simulink library "WBToolboxLibrary"  (R2014b)
settings: Solver=ode45  StartTime=0.0  StopTime=10.0  RelTol=1e-3
undefined symbols (not defined in the file): WBT_modelName, WBT_robotName, WBT_wbiFilename, WBT_wbiList
libraries: simulink x1
(part 1 of 2)
settings Model: CovSaveCumulativeToWorkspaceVar=on  Creator=jorhabib  LastModifiedBy=dferigo

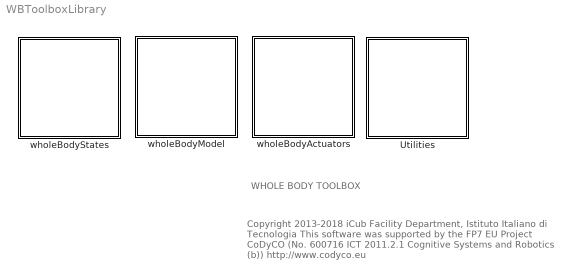
== system WBToolboxLibrary ==
  note: WHOLE BODY TOOLBOX
  note: Copyright  2013-2018 iCub Facility Department, Istituto Italiano di Tecnologia
      | This software was supported by the FP7 EU Project CoDyCO (No. 600716 ICT 2011.2.1 Cognitive Systems and Robotics (b))
      | http://www.codyco.eu
  Utilities : Subsystem
      mask Display: image(imread('utilities.png'))
  wholeBodyActuators : Subsystem
      mask Display: image(imread('wholeBodyActuators.png'),'center')
  wholeBodyModel : Subsystem
      mask Display: image(imread('wholeBodyModel.png'),'center')
  wholeBodyStates : Subsystem
      mask Display: image(imread('wholeBodyStates.png'),'center');

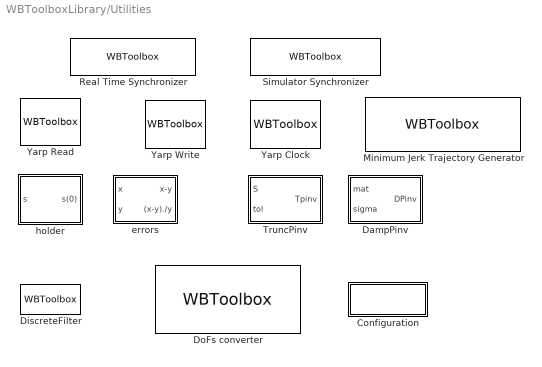
== system WBToolboxLibrary/Utilities ==
  Configuration : Subsystem  InitFcn=|  mask{ConfigSource=Mask, ConfigObject='WBTConfigRobot', RobotName='icub', UrdfFile='model.urdf', ControlledJoints={'l_elbow','l_shoulder_pitch','torso_roll'}, ControlBoardsNames={'left_arm','right_arm','torso'}, LocalName='WBT', GravityVector=[0,0,-9.81]}
      | source = get_param(gcb,'ConfigSource');
      | 
      | if strcmp(source, 'Workspace')
      |     object = get_param(gcb,'ConfigObject');
      |     WBToolbox.ConfigurationToMask(gcb, object);
      | end
      | 
      | WBToolbox.MaskToConfiguration(gcb);
      | 
      | clear object source
      mask prompts: ConfigSource "Configuration from"; ConfigObject "Name of the object"; RobotName "Robot Name"; UrdfFile "Urdf File"; ControlledJoints "Controlled Joints"; ControlBoardsNames "Control Boards Names"; LocalName "Local Name"; GravityVector "Gravity Vector"
      mask TypeOptions ConfigSource: Workspace | Mask
      mask Callback ConfigSource:
      | % Get the Workspace/Mask menu
      | h = Simulink.Mask.get(gcb);
      | currentConfigSource = get_param(gcb,'ConfigSource');
      | 
      | if strcmp(currentConfigSource,'Workspace')
      |     % Switch the visibility of the GUI elements
      |     set_param(gcb,'MaskVisibilities',{'on';'on';'on';'on';'on';'on';'on';'on';});
      |     h.Parameters(3).ReadOnly = 'on';
      |     h.Parameters(4).ReadOnly = 'on';
      |     h.Parameters(5).ReadOnly = 'on';
      |     h.Parameters(6).ReadOnly = 'on';
      |     h.Parameters(7).ReadOnly = 'on';
      |     h.Parameters(8).ReadOnly = 'on';
      | 
      |     % Parse the object inserted in the ConfigObject field
      |     currentConfigObject = get_param(gcb,'ConfigObject');
      |     WBToolbox.ConfigurationToMask(gcb,currentConfigObject);
      |     clear currentConfigObject;
      | elseif strcmp(currentConfigSource,'Mask')
      |     % Switch the visibility of the GUI elements
      |     set_param(gcb,'MaskVisibilities',{'on';'off';'on';'on';'on';'on';'on';'on';});
      |     h.Parameters(3).ReadOnly = 'off';
      |     h.Parameters(4).ReadOnly = 'off';
      |     h.Parameters(5).ReadOnly = 'off';
      |     h.Parameters(6).ReadOnly = 'off';
      |     h.Parameters(7).ReadOnly = 'off';
      |     h.Parameters(8).ReadOnly = 'off';
      |     h.Parameters(3).Enabled = 'on';
      |     h.Parameters(4).Enabled = 'on';
      |     h.Parameters(5).Enabled = 'on';
      |     h.Parameters(6).Enabled = 'on';
      |     h.Parameters(7).Enabled = 'on';
      |     h.Parameters(8).Enabled = 'on';
      | end
      | 
      | clear h currentConfigSource
      mask Callback ConfigObject:
      | % This code get called whatsoever
      | if strcmp(char(get_param(gcb,'ConfigSource')),'Mask')
      |     return
      | end
      | 
      | % Parse the object inserted in the ConfigObject field
      | currentConfigObject = get_param(gcb,'ConfigObject');
      | WBToolbox.ConfigurationToMask(gcb,currentConfigObject);
      | 
      | clear currentConfigObject;
      mask Display: disp('Config')
  DampPinv : Subsystem  mask{tol=1e-4}
      mask prompts: tol "Tolerance"
  DiscreteFilter : S-Function  FunctionName=WBToolbox  Parameters='DiscreteFilter',filterType,numCoeffs,denCoeffs,Fc,Ts,orderMedianFilter,y0,u0  SFunctionDeploymentMode=off  EnableBusSupport=off  mask(Discrete Filter){filterType=Generic, numCoeffs=[0], denCoeffs=[0], Fc=0, Ts=0, orderMedianFilter=0, initStatus=off, y0=[0], u0=[0]}
      mask prompts: filterType "Type of the filter"; numCoeffs "Numerator Coefficients*"; denCoeffs "Denominator Coefficients*"; Fc "Cut Frequency (Hz)"; Ts "Sampling time (s)"; orderMedianFilter "Order"; initStatus "Define initial conditions"; y0 "Output y0"; u0 "Input u0"
      mask help: This block wraps the Filter, FirstOrderLowPassFilter, and MedianFilter from iCub::ctrl.
      mask init:
      | filterType = get_param(gcb, 'filterType');
      | numCoeffs  = mat2str(numCoeffs);
      | denCoeffs  = mat2str(denCoeffs);
      | 
      | initStatus = get_param(gcb, 'initStatus');
      | 
      | if (strcmp(initStatus,'on'))
      |     y0 = mat2str(y0);
      |     u0 = mat2str(u0);
      | else
      |     y0 = 'none';
      |     u0 = 'none';
      | end
      | 
      | clear initStatus
      mask TypeOptions filterType: Generic | FirstOrderLowPassFilter | MedianFilter
      mask Callback filterType:
      | % From: https://it.mathworks.com/help/simulink/slref/simulink.mask-class.html
      | filterType = get_param(gcb, 'filterType');
      | initStatus = get_param(gcb, 'initStatus');
      | p = Simulink.Mask.get(gcbh);
      | howToCoeffs = p.getDialogControl('howToCoeffs');
      | 
      | %set_param(gcb, 'initStatus','off');
      | if (strcmp(initStatus,'on'))
      |     vis_init = 'on';
      | else
      |     vis_init = 'off';
      | end
      | 
      | if(strcmp(filterType, 'Generic'))
      |     set_param(gcb, 'MaskVisibilities',{'on','on','on','off','off','off','on',vis_init,vis_init});
      |     howToCoeffs.Visible = 'on';
      | elseif(strcmp(filterType, 'FirstOrderLowPassFilter'))
      |     set_param(gcb, 'MaskVisibilities',{'on','off','off','on','on','off','on',vis_init,'off'});
      |     howToCoeffs.Visible = 'off';
      | elseif(strcmp(filterType, 'MedianFilter'))
      |     set_param(gcb, 'MaskVisibilities',{'on','off','off','off','off','on','on',vis_init,'off'});
      |     howToCoeffs.Visible = 'off';
      | end
      | 
      | clear filterType initStatus p howToCoeffs vis_init;
      mask Callback initStatus:
      | initStatus   = get_param(gcb, 'initStatus');
      | visibilities = get_param(gcb, 'MaskVisibilities');
      | filterType   = get_param(gcb, 'filterType');
      | 
      | if (strcmp(initStatus,'off'))
      |     visibilities{8} = 'off';
      |     visibilities{9} = 'off';
      | elseif (strcmp(initStatus,'on'))
      |     visibilities{8} = 'on';
      |     if (strcmp(filterType,'Generic'))
      |         visibilities{9} = 'on';
      |     end
      | end
      | 
      | set_param(gcb, 'MaskVisibilities', visibilities);
      | 
      | clear initStatus visibilities filterType;
      mask DialogControl howToCoeffs Prompt: * The coefficients are ordered in increasing power of z^-1
      mask Display: disp('Filter')
  DoFs converter : S-Function  FunctionName=WBToolbox  Parameters='ModelPartitioner',WBTConfigParameters,configBlockAbsName,yarp2WBI  SFunctionDeploymentMode=off  EnableBusSupport=off  mask(DoFs converter){yarp2WBIOption=From YARP to WBI}
      mask prompts: yarp2WBIOption "Conversion Direction"
      mask help:
      | This block converts from a DoFs serialization to a YARP serialization or viceversa depending on its configuration.
      | The robot name is taken from the environment variable YARP_ROBOT_NAME.
      |
      | Parameters:
      |
      | - Conversion direction: specify if you want to convert from YARP to the current DoFs serialization or viceversa.
      mask init:
      | % WBBlock Initialization
      | % ======================
      | 
      | try
      |     [configBlockAbsName, WBTConfig] = WBToolbox.BlockInitialization(gcb, gcs);
      |     
      |     WBTConfigParameters = WBTConfig.getSimulinkParameters;
      |     clear WBTConfig;
      | catch
      | end
      | 
      | % ModelPartitioner Initialization
      | % ===============================
      | 
      | switch get_param(gcb, 'yarp2WBIOption')
      |     case 'From YARP to WBI'
      |         yarp2WBI = true;
      |     case 'From WBI to YARP'
      |         yarp2WBI = false;
      |     otherwise
      | end
      mask TypeOptions yarp2WBIOption: From YARP to WBI | From WBI to YARP
      mask DialogControl toggleHighlighting Prompt: Toggle Config Block Highlighting
      mask DialogControl toggleHighlighting Callback:
      | [configBlock, ~] = WBToolbox.BlockInitialization(gcb, gcs);
      | 
      | try
      |     if (strcmp(get_param(configBlock,'HiliteAncestors'),'none'))
      |         hilite_system(configBlock,'find');
      |     else
      |         hilite_system(configBlock,'none');
      |     end
      | catch
      |     error('[%s:ShowConfigBlock:Callback] Failed to process config block name: %s',gcb,configBlock);
      | end
      | 
      | clear configBlock
      mask Display:
      | robotName = getenv('YARP_ROBOT_NAME');
      | 
      | currentSelection = get_param(gcb,'yarp2WBIoption');
      | 
      | if strcmp(currentSelection,'From YARP to WBI')
      |     direction = 'YARP -> DoFs';
      | else
      |     direction = 'DoFs -> YARP';
      | end
      | 
      | fprintf('%s\n\n%s', robotName, direction);
  Minimum Jerk Trajectory Generator : S-Function  FunctionName=WBToolbox  Parameters='MinimumJerkTrajectoryGenerator',sampleTime, settlingTime, firstDerivatives, secondDerivatives, explicitInitialValue, externalSettlingTime,resetOnSettlingTime  SFunctionDeploymentMode=off  EnableBusSupport=off  mask(Minimum Jerk Trajectory Generator){externalSettlingTime=off, settlingTime=3, sampleTime=0.01, resetOnSettlingTime=off, firstDerivatives=on, secondDerivatives=on, explicitInitialValue=off}
      mask prompts: externalSettlingTime "External Settling Time"; settlingTime "Settling Time"; sampleTime "Sample Time"; resetOnSettlingTime "Reset on Settling Time Changes"; firstDerivatives "Output First Derivative"; secondDerivatives "Output Second Derivative"; explicitInitialValue "Explicit Initial Value"
      mask help:
      | This block wraps the minJerkTrajGen class from iCub::ctrl::minJerkTrajGen.
      |
      | The Minimum Jerk Trajectory Generator is approximated using a
      | 3rd order LTI dynamical system
      | (for more details see [1]).
      | Position, velocity and acceleration trajectories are computed.
      |  The main advantage with respect to the standard polynomial
      | form is that if the reference value yd changes
      | there is no need to recompute the filter coefficients.
      |
      | [1] Pattacini, U.; Nori, F.; Natale, L.; Metta, G.; Sandini, G., "An experimental evaluation of a novel minimum-jerk cartesian controller for humanoid robots," in Intelligent Robots and Systems (IROS), 2010 IEEE/RSJ International Conference on , vol., no., pp.1668-1674, 18-22 Oct. 2010
      | doi: 10.1109/IROS.2010.5650851
      | URL: http://ieeexplore.ieee.org/stamp/stamp.jsp?tp=&arnumber=5650851&isnumber=5648787
      mask Callback externalSettlingTime:
      | externalSettlingTime = get_param(gcb, 'externalSettlingTime');
      | visibility = get_param(gcb, 'MaskVisibilities');
      | if(strcmp(externalSettlingTime, 'on'))
      |     visibility{2} = 'off';
      |     visibility{4} = 'on';
      | else
      |     visibility{2} = 'on';
      |     visibility{4} = 'off';
      | end
      | set_param(gcb, 'MaskVisibilities',visibility);
      | clear externalSettlingTime
      mask Display:
      | firstDer = get_param(gcb, 'firstDerivatives');
      | secondDer = get_param(gcb, 'secondDerivatives');
      | initialValues = get_param(gcb, 'explicitInitialValue');
      | externalSettlingTimeParam = get_param(gcb, 'externalSettlingTime');
      | 
      | %Inputs
      | portIndex = 2;
      | port_label('input', 1, 'Reference')
      | if(strcmp(initialValues, 'on'))
      |     port_label('input', portIndex, 'Initial Value')
      |     portIndex = portIndex + 1;
      | end
      | 
      | if(strcmp(externalSettlingTimeParam, 'on'))
      |     port_label('input', portIndex, 'Settling Time')
      |     portIndex = portIndex + 1;
      | end
      | 
      | %Outputs
      | port_label('output', 1, 'Signal')
      | secondDerPortIndex = 2;
      | if(strcmp(firstDer, 'on'))
      |     port_label('output', 2, 'First Derivative')
      |     secondDerPortIndex = secondDerPortIndex + 1;
      | end
      | if(strcmp(secondDer, 'on'))
      |     port_label('output', secondDerPortIndex, 'Second Derivative')
      | end
  Real Time Synchronizer : S-Function  FunctionName=WBToolbox  Parameters='RealTimeSynchronizer',period  SFunctionDeploymentMode=off  EnableBusSupport=off  mask(Real Time Synchronizer){period=0.01}
      mask prompts: period "Controller Period (in seconds)"
      mask help:
      | This block slows down the simulation trying to match the period specified
      | as parameter (in seconds).
      | The bigger the period the more probable
      | is that Simulink can remain synched with it.
      mask Display: disp('Real Time Synchronizer')
  Simulator Synchronizer : S-Function  FunctionName=WBToolbox  Parameters='SimulatorSynchronizer',period, serverPortName, clientPortName  SFunctionDeploymentMode=off  EnableBusSupport=off  mask(Simulator Synchronizer){period=0.01, serverPortName='/clock/rpc', clientPortName='/WBT_synchronizer/rpc:o'}
      mask prompts: period "Controller Period (in seconds)"; serverPortName "Server Port Name"; clientPortName "Client Port Name"
      mask help:
      | This block synchronizes with the external simulation on a simulator
      | (only Gazebo is supported at the moment).
      mask Display: disp('Simulator Synchronizer')
  TruncPinv : Subsystem  mask{tol=1e-4}
      mask prompts: tol "Tolerance"
  Yarp Clock : S-Function  FunctionName=WBToolbox  Parameters='YarpClock'  SFunctionDeploymentMode=off  EnableBusSupport=off  mask(YARP Clock){}
      mask help:
      | This block outputs the current YARP Time.
      | In a nutshell, this block outputs the equivalent of the C++ function call yarp::os::Time::now()
      mask Display: disp('YARP Time')
  Yarp Read : S-Function  FunctionName=WBToolbox  Parameters='YarpRead',portName,signalSize,blocking,timestamp,autoconnect,errorOnConnection,timeout  SFunctionDeploymentMode=off  EnableBusSupport=off  mask(YARP Read){portName='/portname', signalSize=1, timeout=0.5, blocking=off, timestamp=on, autoconnect=on, errorOnConnection=on}
      mask prompts: portName "Source Port Name"; signalSize "Port Size"; blocking "Blocking Read"; timestamp "Read Timestamp"; errorOnConnection "Error on missing connection"
      mask help:
      | This block behaves as the command 'yarp read'.
      |
      | By default it has the option 'Autoconnect' active, which means that the user can only specify the name of the port ('Source Port Name') from which readings are desired, along with the size of the expected data (e.g. 3 when reading the torso state).
      |
      | When the user unchecks 'Autoconnect', 'Opened Port Name' field shows up and it corresponds to the name of the port the block will create. No autoconnection is performed, and the output will be always zero until the user connects it to some other port from command line using 'yarp connect [from] [dest]'.
      |
      | When 'Autoconnect' is off, an additional output called 'signal' is added to the block. It outputs 1 if the port has received at least one sample, or 0 otherwise.
      mask Callback blocking:
      | blocking_val = get_param(gcb, 'blocking');
      | mask_visibility = get_param(gcb, 'MaskVisibilities');
      | 
      | if(strcmp(blocking_val, 'on'))
      |     mask_visibility{3} = 'on';
      |     set_param(gcb, 'MaskVisibilities', mask_visibility);
      | else
      |     mask_visibility{3} = 'off';
      |     set_param(gcb, 'MaskVisibilities', mask_visibility);
      | end
      | 
      | clear blocking_val mask_visibility
      mask Callback autoconnect:
      | autoconnect_val = get_param(gcb, 'Autoconnect');
      | prompt_string = get_param(gcb, 'MaskPrompts');
      | mask_visibilities = get_param(gcb, 'MaskVisibilities');
      | 
      | if(strcmp(autoconnect_val, 'on'))
      |     prompt_string{1} = 'Source Port Name';
      |     mask_visibilities{7} = 'on';
      |     set_param(gcb, 'MaskVisibilities',mask_visibilities);
      | else
      |     prompt_string{1} = 'Opened Port Name';
      |     mask_visibilities{7} = 'off';
      |     set_param(gcb, 'MaskVisibilities',mask_visibilities);
      | end
      | set_param(gcb, 'MaskPrompts', prompt_string);
      | clear autoconnect_val prompt_string mask_visibilities
      mask Display:
      | port_label('output', 1, 'signal');
      | portNumber = 1;
      | if (timestamp)
      |     portNumber = portNumber + 1;
      |     port_label('output', portNumber, 'timestamp');
      | end
      | 
      | if (~autoconnect)
      |     portNumber = portNumber + 1;
      |     port_label('output', portNumber, 'status');
      | end
  Yarp Write : S-Function  FunctionName=WBToolbox  Parameters='YarpWrite',portName,autoconnect,errorOnConnection  SFunctionDeploymentMode=off  EnableBusSupport=off  mask(YARP Write){portName='/portname', autoconnect=off, errorOnConnection=on}
      mask prompts: portName "Opened Port Name"; errorOnConnection "Error on missing connection"
      mask help:
      | This block behaves as the command 'yarp write'.
      |
      | By default this block opens a port names as the "Opened Port Name" parameter
      | and stream the input signal to that port.
      | If the option "Autoconnect" is specified, the first parameter become the
      | name of the target port to which the data will be stramed,
      | e.g. like "yarp write ... /destinationPort"
      mask Callback autoconnect:
      | autoconnect_val = get_param(gcb, 'Autoconnect');
      | prompt_string = get_param(gcb, 'MaskPrompts');
      | if(strcmp(autoconnect_val, 'on'))
      |     prompt_string{1} = 'Destination Port Name';
      |     set_param(gcb, 'MaskVisibilities',{'on';'on';'on'});
      | else
      |     prompt_string{1} = 'Opened Port Name';
      |     set_param(gcb, 'MaskVisibilities',{'on';'on';'off'});
      | end
      | set_param(gcb, 'MaskPrompts', prompt_string);
      | clear autoconnect_val prompt_string
      mask Display: disp('Yarp Write')
  errors : Subsystem  mask(Errors){}
      mask help:
      | Computes two kinds of errors. The first is just the difference between x
      | and y while the second is the ratio (x-y)/y.
  "holder " : Subsystem  mask(Holder){}
      mask help: This block holds the first input value during the simulation.

== system WBToolboxLibrary/wholeBodyActuators ==
  Set LowLevel PIDs : Subsystem  mask(Set Low Level PIDs){WBTPIDConfigObjectName='', pidType=Position}
      mask prompts: WBTPIDConfigObjectName "WBTPIDConfig Object Name"; pidType "PID Type"
      mask help:
      | This block sets the low level PID values of the controlled joints.
      |
      | The PIDs can be stored in a WBToolbox.PIDConfiguration object, each of them constructed from the WBToolbox.PID class.
      | If the number of PIDs does not match the DoFs of the Configuration block pointed by this SetLowLevelPID block, the default values are used.
      |
      | Parameters:
      | - WBToolbox.PIDConfiguration Object Name: The name of the object which store the PIDs. It must be loaded in the workspace before the simulation runs
      | - PID Type: the type of the target PIDs to set
      mask init:
      | % WBBlock Initialization
      | % ======================
      | 
      | try
      |     [configBlockAbsName, WBTConfig] = WBToolbox.BlockInitialization(gcb, gcs);
      |     
      |     WBTConfigParameters = WBTConfig.getSimulinkParameters;
      |     clear WBTConfig;
      | catch
      | end
      | 
      | % SetLowLevelPIDs Initialization
      | % ==============================
      | 
      | try
      |     PIDObjectName = WBTPIDConfigObjectName;
      |    
      |     % Remove the apices if present
      |     if (PIDObjectName(1) == "'" && ...
      |         PIDObjectName(end) == "'")
      |         PIDObjectName = PIDObjectName(2:end-1);
      |     end
      | 
      |     % Get the struct from the class
      |     PIDs = evalin('base', PIDObjectName);
      |     if (isa(PIDs,'WBToolbox.PIDConfiguration'))
      |         WBTPIDConfigStruct = PIDs.getSimulinkParameters;
      |     end
      | end
      mask TypeOptions pidType: Position | Torque
      mask Callback pidType:
      | % Get the mask parameter values. This is a cell
      | %   array of strings.
      | maskStr = get_param(gcb,'pidType');
      | 
      | switch maskStr
      |     case 'Position'
      |         set_param(gcb,'BackgroundColor', '[0.5137, 0.8510, 0.6706, 1.0]');
      |     case 'Position Direct'
      |         set_param(gcb,'BackgroundColor', '[0.3922, 0.7882, 0.3451, 1.0]');
      |     case 'Velocity'
      |         set_param(gcb,'BackgroundColor', '[0.5137, 0.6745, 1.0000, 1.0]');
      |     case 'Torque'
      |         set_param(gcb,'BackgroundColor', '[0.8275, 0.5765, 0.6039, 1.0]');
      |     otherwise
      |         error('PID Type not recognized');
      | end
      | 
      | clear  maskStr
      mask DialogControl toggleHighlighting Prompt: Toggle Config Block Highlighting
      mask DialogControl toggleHighlighting Callback:
      | [configBlock, ~] = WBToolbox.BlockInitialization(gcb, gcs);
      | 
      | try
      |     if (strcmp(get_param(configBlock,'HiliteAncestors'),'none'))
      |         hilite_system(configBlock,'find');
      |     else
      |         hilite_system(configBlock,'none');
      |     end
      | catch
      |     error('[%s:ShowConfigBlock:Callback] Failed to process config block name: %s',gcb,configBlock);
      | end
      | 
      | clear configBlock
      mask Display:
      | pidType = get_param(gcb,'pidType');
      | description = sprintf('Set Low Level\n%s PIDs', pidType);
      | disp(description);
  Set References : Subsystem  mask(Set References){controlType=Position, refSpeed=50}
      mask prompts: controlType "Control Mode"; refSpeed "Reference Speed"
      mask help:
      | This block sets the references for the robot actuators.
      | The type of control mode is specified as a parameter in the block.
      |
      | Assuming DoFs is the number of degrees of freedom configured in the Config block associated:
      |
      | Input:
      | - References: Vector of size DoFs, representing the references to be sent to the robot controlled joints.
      | - Reference Speed (Position): Set the reference speed used by the trajectory generator of the IPositionControl interface
      |
      | Parameters:
      | - Control Mode: The control mode. Choose one of the supplied mode.
      mask init:
      | % WBBlock Initialization
      | % ======================
      | 
      | try
      |     [configBlockAbsName, WBTConfig] = WBToolbox.BlockInitialization(gcb, gcs);
      |     
      |     WBTConfigParameters = WBTConfig.getSimulinkParameters;
      |     clear WBTConfig;
      | catch
      | end
      mask TypeOptions controlType: Position | Position Direct | Velocity | Torque | Open Loop | PWM | Current
      mask Callback controlType:
      | % Get the mask parameter values. This is a cell
      | %   array of strings.
      | 
      | maskStr = get_param(gcb,'controlType');
      | 
      | switch maskStr
      |     case 'Position'
      |         set_param(gcb,'BackgroundColor', '[0.5137, 0.8510, 0.6706, 1.0]');
      |         set_param(gcb,'MaskVisibilities', {'on';'on'});
      |     case 'Position Direct'
      |         set_param(gcb,'BackgroundColor', '[0.3922, 0.7882, 0.3451, 1.0]');
      |         set_param(gcb,'MaskVisibilities', {'on';'off'});
      |     case 'Velocity'
      |         set_param(gcb,'BackgroundColor', '[0.5137, 0.6745, 1.0000, 1.0]');
      |         set_param(gcb,'MaskVisibilities', {'on';'off'});
      |     case 'Torque'
      |         set_param(gcb,'BackgroundColor', '[0.8275, 0.5765, 0.6039, 1.0]');
      |         set_param(gcb,'MaskVisibilities', {'on';'off'});
      |     case 'Open Loop'
      |         set_param(gcb,'BackgroundColor', '[0.98, 0.98, 0.98, 1.0]');
      |         set_param(gcb,'MaskVisibilities', {'on';'off'});
      |     case 'PWM'
      |         set_param(gcb,'BackgroundColor', '[1, 1, 1, 1.0]');
      |         set_param(gcb,'MaskVisibilities', {'on';'off'});
      |     case 'Current'
      |         set_param(gcb,'BackgroundColor', '[0.96, 0.77, 0.46, 1.0]');
      |         set_param(gcb,'MaskVisibilities', {'on';'off'});
      |     otherwise
      |         error('Control Type not recognized.')
      | end
      | 
      | clear  maskStr
      mask DialogControl toggleHighlighting Prompt: Toggle Config Block Highlighting
      mask DialogControl toggleHighlighting Callback:
      | [configBlock, ~] = WBToolbox.BlockInitialization(gcb, gcs);
      | 
      | try
      |     if (strcmp(get_param(configBlock,'HiliteAncestors'),'none'))
      |         hilite_system(configBlock,'find');
      |     else
      |         hilite_system(configBlock,'none');
      |     end
      | catch
      |     error('[%s:ShowConfigBlock:Callback] Failed to process config block name: %s',gcb,configBlock);
      | end
      | 
      | clear configBlock
      mask Display:
      | disp(get_param(gcb,'controlType'))
      | %port_label('input',1,'References')

== system WBToolboxLibrary/wholeBodyModel ==
  Dynamics : Subsystem
      mask Display: image(imread('Dynamics.png'))
  Jacobians : Subsystem
      mask Display: image(imread('jacobian.png'))
  Kinematics : Subsystem
      mask Display: image(imread('forwardKinematics.png'))

== system WBToolboxLibrary/wholeBodyStates ==
  Get Limits : Subsystem  mask(Get Limits){limitsSource=ControlBoard, limitsType=Position}
      mask prompts: limitsSource "Limits Source"; limitsType "Limits Type"
      mask help:
      | This block provides the joint limits gathering data from either the Robot's Control Board or URDF model.
      |
      | Output:
      |
      | * Max: 1xDoFs vector containing the maximum limit
      | * Min:  1xDoFs vector containing the maximum limit
      |
      | Measures are in radians.
      mask init:
      | % WBBlock Initialization
      | % ======================
      | 
      | try
      |     [configBlockAbsName, WBTConfig] = WBToolbox.BlockInitialization(gcb, gcs);
      |     
      |     WBTConfigParameters = WBTConfig.getSimulinkParameters;
      |     clear WBTConfig;
      | catch
      | end
      | 
      | % GetLimits Initialization
      | % =========================
      | 
      | sourceLimit = get_param(gcb,'limitsSource');
      | typeLimit = get_param(gcb,'limitsType');
      | notifyError = false;
      | 
      | switch sourceLimit
      |     case 'ControlBoard'
      |         switch typeLimit
      |             case 'Position'
      |                 limitsType = 'ControlBoardPosition';
      |             case 'Velocity'
      |                 limitsType = 'ControlBoardVelocity';
      |             otherwise
      |                 notifyError = true;
      |         end
      |     case 'URDF'
      |         switch typeLimit
      |             case 'Position'
      |                 limitsType = 'ModelPosition';
      |             otherwise
      |                 notifyError = true;
      |         end
      | end
      | 
      | if notifyError
      |     error('Limit Type not recognized');
      | end
      | 
      | clear sourceLimit typeLimit notifyError
      mask TypeOptions limitsSource: ControlBoard | URDF
      mask Callback limitsSource:
      | sourceLimit = get_param(gcb,'limitsSource');
      | blockParameters = Simulink.Mask.get(gcb).Parameters;
      | limitsTypeBlockParam = blockParameters(2);
      | 
      | switch sourceLimit
      |     case 'ControlBoard'
      |         limitsTypeBlockParam.TypeOptions = {'Position','Velocity'};
      |         %limitsTypeBlockParam.Value = limitsTypeBlockParam.TypeOptions{1};
      |     case 'URDF'
      |         limitsTypeBlockParam.TypeOptions = {'Position'};
      |         %limitsTypeBlockParam.Value = limitsTypeBlockParam.TypeOptions{1};
      |     otherwise
      |         error('Limit Source not recognized');
      | end
      | 
      | clear sourceLimit blockParameters limitsTypeBlockParam
      mask TypeOptions limitsType: Position | Velocity
      mask Callback limitsType:
      | % Get the mask parameter values. This is a cell array of strings.
      | %
      | maskStr = get_param(gcb,'limitsType');
      | if strcmp(maskStr, 'Position')
      |     set_param(gcb,'BackgroundColor', '[0.5137, 0.8510, 0.6706, 1.0]');
      | elseif strcmp(maskStr, 'Velocity')
      |     set_param(gcb,'BackgroundColor', '[0.5137, 0.6745, 1.0000, 1.0]');
      | elseif strcmp(maskStr, 'Acceleration')
      |     set_param(gcb,'BackgroundColor', '[0.9255, 0.8706, 0.1333, 1.0]');
      | elseif strcmp(maskStr, 'Torque')
      |     set_param(gcb,'BackgroundColor', '[0.8275, 0.5765, 0.6039, 1.0]');
      | end
      | clear  maskStr
      mask DialogControl toggleHighlighting Prompt: Toggle Config Block Highlighting
      mask DialogControl toggleHighlighting Callback:
      | [configBlock, ~] = WBToolbox.BlockInitialization(gcb, gcs);
      | 
      | try
      |     if (strcmp(get_param(configBlock,'HiliteAncestors'),'none'))
      |         hilite_system(configBlock,'find');
      |     else
      |         hilite_system(configBlock,'none');
      |     end
      | catch
      |     error('[%s:ShowConfigBlock:Callback] Failed to process config block name: %s',gcb,configBlock);
      | end
      | 
      | clear configBlock
      mask Display:
      | fprintf('%s\n(%s)',get_param(gcb,'limitsType'),get_param(gcb,'limitsSource'))
      | 
      | port_label('output',1,'Min')
      | port_label('output',2,'Max')
  Get Measurement : Subsystem  mask(Get Measurement){measuredType=Joints Position}
      mask prompts: measuredType "Estimate Type"
      mask help:
      | This block gathers the measurement of the specified type.
      |
      | Assuming DoFs is the number of degrees of freedom of the robot,
      |
      | Output:
      | * References: Vector of size DoFs, representing the requested measurement.
      |
      | Parameters:
      | * Control Mode: The control mode. Choose one of the supplied mode.
      mask init: same as WBToolboxLibrary/wholeBodyActuators/Set References
      mask TypeOptions measuredType: Joints Position | Joints Velocity | Joints Acceleration | Joints Torque
      mask Callback measuredType:
      | % Get the mask parameter values. This is a cell
      | %   array of strings.
      | 
      | maskStr = get_param(gcb,'measuredType');
      | if strcmp(maskStr, 'Joints Position')
      |     set_param(gcb,'BackgroundColor', '[0.5137, 0.8510, 0.6706, 1.0]');
      | elseif strcmp(maskStr, 'Joints Velocity')
      |     set_param(gcb,'BackgroundColor', '[0.5137, 0.6745, 1.0000, 1.0]');
      | elseif strcmp(maskStr, 'Joints Acceleration')
      |     set_param(gcb,'BackgroundColor', '[0.9255, 0.8706, 0.1333, 1.0]');
      | elseif strcmp(maskStr, 'Joints Torque')
      |     set_param(gcb,'BackgroundColor', '[0.8275, 0.5765, 0.6039, 1.0]');
      | end
      | clear  maskStr
      mask DialogControl toggleHighlighting Prompt: Toggle Config Block Highlighting
      mask DialogControl toggleHighlighting Callback:
      | [configBlock, ~] = WBToolbox.BlockInitialization(gcb, gcs);
      | 
      | try
      |     if (strcmp(get_param(configBlock,'HiliteAncestors'),'none'))
      |         hilite_system(configBlock,'find');
      |     else
      |         hilite_system(configBlock,'none');
      |     end
      | catch
      |     error('[%s:ShowConfigBlock:Callback] Failed to process config block name: %s',gcb,configBlock);
      | end
      | 
      | clear configBlock
      mask Display: port_label('output', 1, get_param(gcb,'measuredType'))

== system WBToolboxLibrary/Utilities/Configuration ==
  ImConfig : Constant  Value=0
  Terminator : Terminator
  wires:
  ImConfig/1 -> Terminator/1

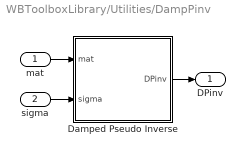
== system WBToolboxLibrary/Utilities/DampPinv ==
  mat : Inport
  sigma : Inport  Port=2
  Damped Pseudo Inverse : MATLAB Function  TreatAsAtomicUnit=on
      settings: PermitHierarchicalResolution=ParametersOnly
  DPinv : Outport
  wires:
  sigma/1 -> Damped Pseudo Inverse/2(sigma)
  Damped Pseudo Inverse/1(DPinv) -> DPinv/1
  mat/1 -> Damped Pseudo Inverse/1(mat)

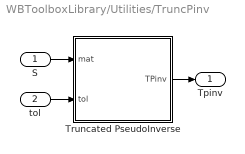
== system WBToolboxLibrary/Utilities/TruncPinv ==
  S : Inport
  tol : Inport  Port=2
  Truncated PseudoInverse : MATLAB Function  TreatAsAtomicUnit=on
      settings: PermitHierarchicalResolution=ParametersOnly
  Tpinv : Outport
  wires:
  S/1 -> Truncated PseudoInverse/1(mat)
  Truncated PseudoInverse/1(TPinv) -> Tpinv/1
  tol/1 -> Truncated PseudoInverse/2(tol)

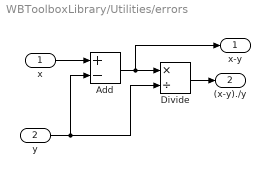
== system WBToolboxLibrary/Utilities/errors ==
  x : Inport
  y : Inport  Port=2
  Add : Sum  Inputs=+-
  Divide : Product  Inputs=*/
  x-y : Outport
  (x-y)./y : Outport  Port=2
  wires:
  Add/1 -> Divide/1, x-y/1
  x/1 -> Add/1
  y/1 -> Add/2, Divide/2
  Divide/1 -> (x-y)./y/1

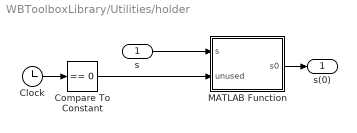
== system WBToolboxLibrary/Utilities/holder  ==
  s : Inport
  Clock : Clock
  Compare To Constant : simulink/Logic and Bit Operations/Compare To Constant  relop===  const=0  OutDataTypeStr=boolean
  MATLAB Function : MATLAB Function  TreatAsAtomicUnit=on
      settings: PermitHierarchicalResolution=ParametersOnly
  s(0) : Outport
  wires:
  Clock/1 -> Compare To Constant/1
  MATLAB Function/1(s0) -> s(0)/1
  s/1 -> MATLAB Function/1(s)
  Compare To Constant/1 -> MATLAB Function/2(unused)

== system WBToolboxLibrary/wholeBodyActuators/Set LowLevel PIDs ==
  S-Function : S-Function  FunctionName=WBToolbox  Parameters='SetLowLevelPID',WBTConfigParameters,configBlockAbsName,WBTPIDConfigStruct,pidType  SFunctionDeploymentMode=off  EnableBusSupport=off

== system WBToolboxLibrary/wholeBodyActuators/Set References ==
  References : Inport
  S-Function : S-Function  FunctionName=WBToolbox  Parameters='SetReferences',WBTConfigParameters,configBlockAbsName,controlType,refSpeed  SFunctionDeploymentMode=off  EnableBusSupport=off
  wires:
  References/1 -> S-Function/1

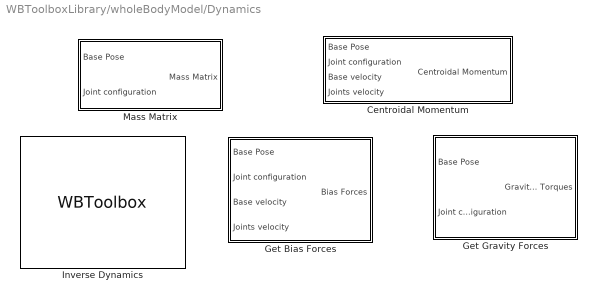
== system WBToolboxLibrary/wholeBodyModel/Dynamics ==
  Centroidal Momentum : Subsystem  mask(Centroidal Momentum){}
      mask help:
      | This block computed the 6 element centroidal momentum, as defined in:
      | "Centroidal dynamics of a humanoid robot" - DE Orin, A Goswami, SH Lee -
      | Autonomous Robots 35 (2-3), 161-176
      |
      | Assuming DoFs is the number of degrees of freedom of the robot:
      |
      | Input:
      | - Base pose: 4x4 matrix representing the homogenous transformation between the base frame and the world frame.
      | - Joint configuration: Vector of size DoFs, representing the configuration of the joints.
      | - Base velocity: Vector of size 6 representing the linear and angular velocity of the base frame.
      | - Joints velocity: Vector of size DoFs, representing the velocity of the joints.
      |
      | Output:
      | - Centroidal Momentum: 6-element vector containg the centroidal momentum (3 value for linear momentum and 3 for angular momentum)
      mask init: same as WBToolboxLibrary/wholeBodyActuators/Set References
      mask DialogControl toggleHighlighting Prompt: Toggle Config Block Highlighting
      mask DialogControl toggleHighlighting Callback:
      | [configBlock, ~] = WBToolbox.BlockInitialization(gcb, gcs);
      | 
      | try
      |     if (strcmp(get_param(configBlock,'HiliteAncestors'),'none'))
      |         hilite_system(configBlock,'find');
      |     else
      |         hilite_system(configBlock,'none');
      |     end
      | catch
      |     error('[%s:ShowConfigBlock:Callback] Failed to process config block name: %s',gcb,configBlock);
      | end
      | 
      | clear configBlock
  Get Bias Forces : Subsystem  mask(Get Generalized Bias Forces){}
      mask help:
      | This block retrieves the generalied bias forces of the robot.
      |
      | Assuming DoFs is the number of degrees of freedom of the robot:
      |
      | Input:
      | - Base pose: 4x4 matrix representing the homogenous transformation between the base frame and the world frame.
      | - Joint configuration: Vector of size DoFs, representing the configuration of the joints.
      | - Base velocity: Vector of size 6 representing the linear and angular velocity of the base frame.
      | - Joints velocity: Vector of size DoFs, representing the velocity of the joints.
      |
      | Output:
      | - Bias Forces: a Dofs + 6 vector representing the generalized bias forces of the robot.
      mask init: same as WBToolboxLibrary/wholeBodyActuators/Set References
      mask DialogControl toggleHighlighting Prompt: Toggle Config Block Highlighting
      mask DialogControl toggleHighlighting Callback:
      | [configBlock, ~] = WBToolbox.BlockInitialization(gcb, gcs);
      | 
      | try
      |     if (strcmp(get_param(configBlock,'HiliteAncestors'),'none'))
      |         hilite_system(configBlock,'find');
      |     else
      |         hilite_system(configBlock,'none');
      |     end
      | catch
      |     error('[%s:ShowConfigBlock:Callback] Failed to process config block name: %s',gcb,configBlock);
      | end
      | 
      | clear configBlock
  Get Gravity Forces : Subsystem  mask(Gravity bias){}
      mask help:
      | This block compute the generalized bias forces due to the gravity
      |
      | Assuming DoFs is the number of degrees of freedom of the robot:
      |
      | Input:
      | - Base pose: 4x4 matrix representing the homogenous transformation between the base frame and the world frame.
      | - Joint configuration: Vector of size DoFs, representing the configuration of the joints.
      |
      | Output:
      | - Gravity: a Dofs + 6 vector representing the torques due to the gravity.
      mask init: same as WBToolboxLibrary/wholeBodyActuators/Set References
      mask DialogControl toggleHighlighting Prompt: Toggle Config Block Highlighting
      mask DialogControl toggleHighlighting Callback:
      | [configBlock, ~] = WBToolbox.BlockInitialization(gcb, gcs);
      | 
      | try
      |     if (strcmp(get_param(configBlock,'HiliteAncestors'),'none'))
      |         hilite_system(configBlock,'find');
      |     else
      |         hilite_system(configBlock,'none');
      |     end
      | catch
      |     error('[%s:ShowConfigBlock:Callback] Failed to process config block name: %s',gcb,configBlock);
      | end
      | 
      | clear configBlock
  Inverse Dynamics : S-Function  FunctionName=WBToolbox  Parameters='InverseDynamics',WBTConfigParameters,configBlockAbsName  SFunctionDeploymentMode=off  EnableBusSupport=off  mask(Inverse Dynamics){}
      mask help:
      | This block compute the inverse dynamics of the robot.
      |
      | Assuming DoFs is the number of degrees of freedom of the robot:
      |
      | Input:
      | - Base pose: 4x4 matrix representing the homogenous transformation between the base frame and the world frame.
      | - Joint configuration: Vector of size DoFs, representing the configuration of the joints.
      | - Base velocity: Vector of size 6 representing the linear and angular velocity of the base frame.
      | - Joints velocity: Vector of size DoFs, representing the velocity of the joints.
      | - Base acceleration: Vector of size 6 representing the linear and angular acceleration of the base frame.
      | - Joints acceleration: Vector of size DoFs, representing the acceleration of the joints.
      |
      | Output:
      | - Torques: a Dofs + 6 vector representing the corresponding torques required to achive the desired accelerations given the robot state
      mask init: same as WBToolboxLibrary/wholeBodyActuators/Set References
      mask DialogControl toggleHighlighting Prompt: Toggle Config Block Highlighting
      mask DialogControl toggleHighlighting Callback:
      | [configBlock, ~] = WBToolbox.BlockInitialization(gcb, gcs);
      | 
      | try
      |     if (strcmp(get_param(configBlock,'HiliteAncestors'),'none'))
      |         hilite_system(configBlock,'find');
      |     else
      |         hilite_system(configBlock,'none');
      |     end
      | catch
      |     error('[%s:ShowConfigBlock:Callback] Failed to process config block name: %s',gcb,configBlock);
      | end
      | 
      | clear configBlock
      mask Display:
      | port_label('output', 1, 'Torques')
      | 
      | port_label('input', 1, 'Base pose')
      | port_label('input', 2, 'Joints configuration')
      | port_label('input', 3, 'Base velocity')
      | port_label('input', 4, 'Joints velocity')
      | port_label('input', 5, 'Base acceleration')
      | port_label('input', 6, 'Joints acceleration')
  Mass Matrix : Subsystem  mask(Mass Matrix){}
      mask help:
      | This block retrieves the robot mass matrix.
      |
      | Assuming DoFs is the number of degrees of freedom of the robot,
      | Input:
      | - Base pose: 4x4 matrix representing the homogenous transformation between the base frame and the world frame.
      | - Joint configuration: Vector of size DoFs, representing the configuration of the joints.
      |
      | Output:
      | - Mass Matrix: a (Dofs + 6) x (Dofs + 6) matrix representing the mass matrix of the robot
      mask init: same as WBToolboxLibrary/wholeBodyActuators/Set References
      mask DialogControl toggleHighlighting Prompt: Toggle Config Block Highlighting
      mask DialogControl toggleHighlighting Callback:
      | [configBlock, ~] = WBToolbox.BlockInitialization(gcb, gcs);
      | 
      | try
      |     if (strcmp(get_param(configBlock,'HiliteAncestors'),'none'))
      |         hilite_system(configBlock,'find');
      |     else
      |         hilite_system(configBlock,'none');
      |     end
      | catch
      |     error('[%s:ShowConfigBlock:Callback] Failed to process config block name: %s',gcb,configBlock);
      | end
      | 
      | clear configBlock

== system WBToolboxLibrary/wholeBodyModel/Jacobians ==
  DotJ Nu : Subsystem  mask(DotJ Nu){frameName='frame'}
      mask prompts: frameName "Frame name"
      mask help:
      | This block computes the product between the time derivative of the Jacobian of the specified frame and the state (base and joints) velocity vector.
      |
      | Assuming DoFs is the number of degrees of freedom of the robot:
      |
      | Input:
      | - Base pose: 4x4 matrix representing the homogenous transformation between the the base frame and the world frame.
      | - Joint configuration: Vector of size DoFs, representing the configuration of the joints.
      | - Base velocity: Vector of size 6 representing the linear and angular velocity of the base frame.
      | - Joints velocity: Vector of size DoFs, representing the velocity of the joints.
      |
      | Output:
      | - dotJ nu: a 6-d vector representing the product between the time derivative of the
      |          Jacobian of the specified frame and the state velocity vector
      |
      | Parameters:
      | - Frame name: the name of the frame. It should be specified in the URDF model.
      mask init: same as WBToolboxLibrary/wholeBodyActuators/Set References
      mask DialogControl toggleHighlighting Prompt: Toggle Config Block Highlighting
      mask DialogControl toggleHighlighting Callback:
      | [configBlock, ~] = WBToolbox.BlockInitialization(gcb, gcs);
      | 
      | try
      |     if (strcmp(get_param(configBlock,'HiliteAncestors'),'none'))
      |         hilite_system(configBlock,'find');
      |     else
      |         hilite_system(configBlock,'none');
      |     end
      | catch
      |     error('[%s:ShowConfigBlock:Callback] Failed to process config block name: %s',gcb,configBlock);
      | end
      | 
      | clear configBlock
      mask Display:
      | escapedFrameName = strrep(frameName, '_', '\_');
      | port_label('output', 1, strcat('dot J_{',escapedFrameName,'} \nu'), 'texmode','on')
      | 
      | port_label('input', 1, '{}^{world} H_{base}', 'texmode','on')
      | port_label('input', 2, 'Joint configuration')
      | port_label('input', 3, 'Base velocity')
      | port_label('input', 4, 'Joint velocity')
      | 
      | clear escapedFrameName;
  Jacobian : Subsystem  mask(Jacobian){frameName='frame'}
      mask prompts: frameName "Frame name"
      mask help:
      | This block retrieves the Jacobian of the specified frame.
      |
      | Assuming DoFs is the number of degrees of freedom of the robot:
      |
      | Input:
      | - Base pose: 4x4 matrix representing the homogenous transformation between the the base frame and the world frame.
      | - Joint configuration: Vector of size DoFs, representing the configuration of the joints.
      |
      | Output:
      | - Jacobian: a 6x6+dofs matrix representing the Jacobian of the specified frame written in the world frame.
      |
      | Parameters:
      | - Frame name: the name of the frame. It should be specified in the URDF model.
      mask init: same as WBToolboxLibrary/wholeBodyActuators/Set References
      mask DialogControl toggleHighlighting Prompt: Toggle Config Block Highlighting
      mask DialogControl toggleHighlighting Callback:
      | [configBlock, ~] = WBToolbox.BlockInitialization(gcb, gcs);
      | 
      | try
      |     if (strcmp(get_param(configBlock,'HiliteAncestors'),'none'))
      |         hilite_system(configBlock,'find');
      |     else
      |         hilite_system(configBlock,'none');
      |     end
      | catch
      |     error('[%s:ShowConfigBlock:Callback] Failed to process config block name: %s',gcb,configBlock);
      | end
      | 
      | clear configBlock
      mask Display:
      | escapedFrameName = strrep(frameName, '_', '\_');
      | port_label('output', 1, strcat('{}^{world} J_{',escapedFrameName,'}'), 'texmode','on')
      | 
      | port_label('input', 1, '{}^{world} H_{base}', 'texmode','on')
      | port_label('input', 2, 'Joint configuration')
      | 
      | clear escapedFrameName;
